simulink model "mKinBlock"  (R2021a)
settings: Solver=VariableStepAuto  StartTime=0.0  StopTime=10.0  RelTol=1e-3
settings Model: Creator=angelo  LastModifiedBy=angelo

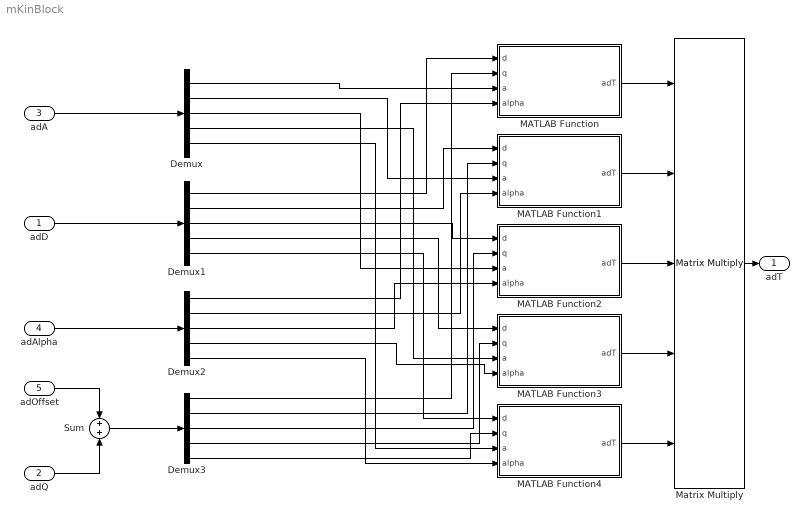
== system mKinBlock ==
  adD : Inport
  adQ : Inport  Port=2
  adA : Inport  Port=3
  adAlpha : Inport  Port=4
  adOffset : Inport  Port=5
  Demux{,1..3} (4 alike) : Demux  Outputs=5
  MATLAB Function : MATLAB Function  TreatAsAtomicUnit=on
  MATLAB Function1 : MATLAB Function  TreatAsAtomicUnit=on
  MATLAB Function2 : MATLAB Function  TreatAsAtomicUnit=on
  MATLAB Function3 : MATLAB Function  TreatAsAtomicUnit=on
  MATLAB Function4 : MATLAB Function  TreatAsAtomicUnit=on
  Matrix Multiply : Product  Inputs=5  Multiplication=Matrix(*)
  Sum : Sum
  adT : Outport
  wires:
  adA/1 -> Demux/1
  adD/1 -> Demux1/1
  adAlpha/1 -> Demux2/1
  Sum/1 -> Demux3/1
  Demux/1 -> MATLAB Function/3(a)
  Demux/2 -> MATLAB Function1/3(a)
  Demux/3 -> MATLAB Function2/3(a)
  Demux/4 -> MATLAB Function3/3(a)
  Demux/5 -> MATLAB Function4/3(a)
  Demux1/1 -> MATLAB Function/1(d)
  Demux1/2 -> MATLAB Function1/1(d)
  Demux1/3 -> MATLAB Function2/1(d)
  Demux1/4 -> MATLAB Function3/1(d)
  Demux1/5 -> MATLAB Function4/1(d)
  Demux2/1 -> MATLAB Function/4(alpha)
  Demux2/2 -> MATLAB Function1/4(alpha)
  Demux2/3 -> MATLAB Function2/4(alpha)
  Demux2/4 -> MATLAB Function3/4(alpha)
  Demux2/5 -> MATLAB Function4/4(alpha)
  Demux3/1 -> MATLAB Function/2(q)
  Demux3/2 -> MATLAB Function1/2(q)
  Demux3/3 -> MATLAB Function2/2(q)
  Demux3/4 -> MATLAB Function3/2(q)
  Demux3/5 -> MATLAB Function4/2(q)
  MATLAB Function2/1(adT) -> Matrix Multiply/3
  MATLAB Function1/1(adT) -> Matrix Multiply/2
  MATLAB Function/1(adT) -> Matrix Multiply/1
  MATLAB Function3/1(adT) -> Matrix Multiply/4
  MATLAB Function4/1(adT) -> Matrix Multiply/5
  adQ/1 -> Sum/2
  adOffset/1 -> Sum/1
  Matrix Multiply/1 -> adT/1

== matlab function mKinBlock/MATLAB Function1 ==
  data: d input; adT output; q input; a input; alpha input
function adT = kin(d, q, a, alpha)
    adT = functions.computeT(d, q, a, alpha);
end

== matlab function mKinBlock/MATLAB Function ==
  data: d input; adT output; q input; a input; alpha input
function adT = kin(d, q, a, alpha)
    adT = functions.computeT(d, q, a, alpha);
end

== matlab function mKinBlock/MATLAB Function2 ==
  data: d input; adT output; q input; a input; alpha input
function adT = kin(d, q, a, alpha)
    adT = functions.computeT(d, q, a, alpha);
end

== matlab function mKinBlock/MATLAB Function3 ==
  data: d input; adT output; q input; a input; alpha input
function adT = kin(d, q, a, alpha)
    adT = functions.computeT(d, q, a, alpha);
end

== matlab function mKinBlock/MATLAB Function4 ==
  data: d input; adT output; q input; a input; alpha input
function adT = kin(d, q, a, alpha)
    adT = functions.computeT(d, q, a, alpha);
end
